simulink model "AUV_PM"  (R2020b)
settings: Solver=VariableStepAuto  StartTime=0.0  StopTime=10.0  RelTol=1e-3
InitFcn:
  | AUV_VehicleParameters
libraries: fl_lib x44, ee_lib x42, nesl_utility x33, AUVPropulsionSSC_lib x2
(part 1 of 2)
settings Model: DataDictionary=SignalInterfacesDD.sldd  Creator=jantonio  LastModifiedBy=jantonio

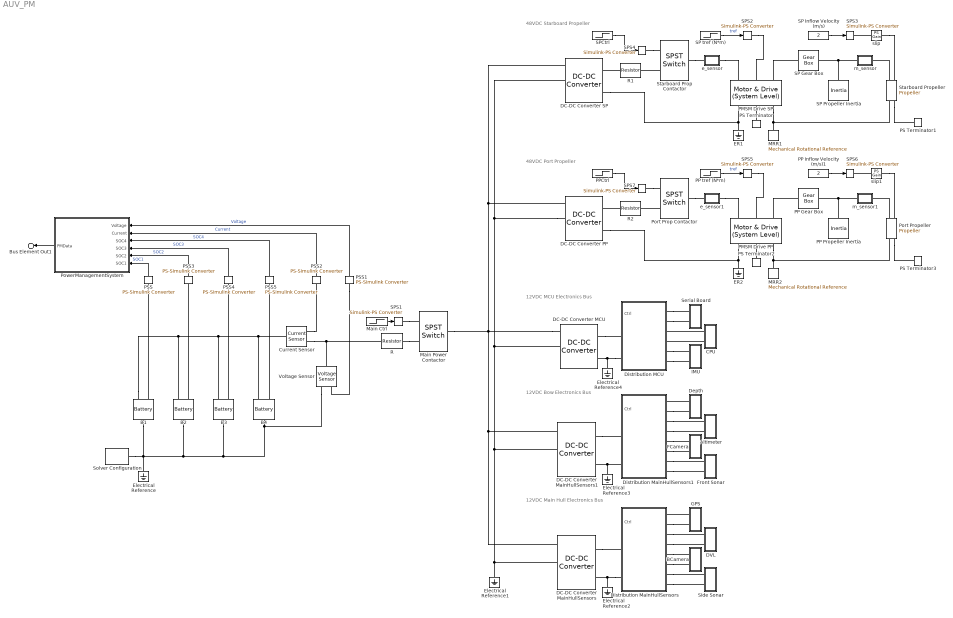
== system AUV_PM ==
  note: 12VDC Bow Electronics Bus
  note: 48VDC Port Propeller
  note: 12VDC MCU Electronics Bus
  note: 48VDC Starboard Propeller
  note: 12VDC Main Hull Electronics Bus
  Altimeter : Subsystem
  B{1..4} (4 alike) : ee_lib/Sources/Battery  Vnom=Vehicle.Battery.voltage V  prm_dir=1  R1_dis=2 Ohm  R1_ch=2 Ohm  R1=Vehicle.Battery.resistance Ohm  prm_AH=2  AH=Vehicle.Battery.capacity hr*A  V1=Vehicle.Battery.v1atAH1 V  AH1=Vehicle.Battery.AH1atV1 hr*A  prm_R2=1  R2=2000 Ohm  prm_dyn=2  Rp1=Vehicle.Battery.R1 Ohm  tau1=Vehicle.Battery.tau1 s  Rp2=0.005 Ohm  tau2=100 s  Rp3=0.005 Ohm  tau3=30 s  Rp4=0.005 Ohm  tau4=30 s  Rp5=0.005 Ohm  tau5=30 s  prm_fade=1  N_fade=100  AH_fade=45 hr*A  R1_fade=2.02 Ohm  R1_ch_fade=2.02 Ohm  V1_fade=10.35 V  i_specify=off  i_priority=None  i=0 A  i_nominal_specify=off  i_nominal_unit=A  i_nominal_value=1  v_specify=off  v_priority=None  v=0 V  v_nominal_specify=off  v_nominal_unit=V  v_nominal_value=1  charge_specify=on  charge_priority=High  charge=Vehicle.Battery.initcapacity hr*A  charge_nominal_specify=off  charge_nominal_unit=hr*A  charge_nominal_value=1  num_cycles_specify=off  num_cycles_priority=High  num_cycles=0  num_cycles_nominal_specify=off  num_cycles_nominal_unit=1  num_cycles_nominal_value=1  thermal_mass=30000 J/K  Tmeas=298.15 K  Vnom_T2=12 V  R1_T2=2.2 Ohm  R1_T2_dis=2.2 Ohm  R1_T2_ch=2.2 Ohm  V1_T2=11.4 V  R2_T2=2200 Ohm  Rp1_T2=0.005 Ohm  tau1_T2=30 s  Rp2_T2=0.005 Ohm  tau2_T2=30 s  Rp3_T2=0.005 Ohm  tau3_T2=30 s  Rp4_T2=0.005 Ohm  tau4_T2=30 s  Rp5_T2=0.005 Ohm  tau5_T2=30 s  Tmeas2=273.15 K  temperature_specify=off  temperature_priority=High  temperature=298.15 K  temperature_nominal_specify=off  temperature_nominal_unit=K  temperature_nominal_value=1
      settings: InternalSimscapePortConfiguration="{\"Bottom\":[],\"Left\":[{\"id\":\"p\",\"label\":\"+\",\"type\":\"foundation.electrical.electrical\"},{\"id\":\"q\",\"label\":\"q\",\"type\":\"output\"}],\"Right\":[{\"id\":\"n\",\"label\":\"-\",\"type\":\"foundation.electrical.electrical\"}],\"Top\":[]}"
  BCamera : Subsystem
  CPU : Subsystem
  Current Sensor : fl_lib/Electrical/Electrical Sensors/Current Sensor
  DC-DC Converter MCU : ee_lib/Semiconductors & Converters/Converters/DC-DC Converter  Vref_option=ee.enum.converters.voltageref.internal  v_ref=10 V  P_rated=10 W  droop_param=1  droop=0.1 V/A  droop_percent=2  reversible=0  efficiency=80  P_fixed=1 W  model_dynamics=0  tau=0.02 s  v_ini=10 V  G_diode=1e-8 1/Ohm  i1_max=2 A  fault_condition=1  fault_threshold=0.5  thermal_mass=100 J/K  initial_temperature=298.15 K
      settings: SourceProductBaseCode=PS  InternalSimscapePortConfiguration="{\"Bottom\":[],\"Left\":[{\"id\":\"p1\",\"label\":\"1+\",\"type\":\"foundation.electrical.electrical\"},{\"id\":\"n1\",\"label\":\"1-\",\"type\":\"foundation.electrical.electrical\"},{\"id\":\"F\",\"label\":\"F\",\"type\":\"input\"}],\"Right\":[{\"id\":\"p2\",\"label\":\"2+\",\"type\":\"foundation.electrical.electrical\"},{\"id\":\"n2\",\"label\":\"2-\",\"type\":\"foundation.electrical.electrical\"}],\"Top\":[]}"
  DC-DC Converter MainHullSensors : ee_lib/Semiconductors & Converters/Converters/DC-DC Converter  Vref_option=ee.enum.converters.voltageref.internal  v_ref=10 V  P_rated=10 W  droop_param=1  droop=0.1 V/A  droop_percent=2  reversible=0  efficiency=80  P_fixed=1 W  model_dynamics=0  tau=0.02 s  v_ini=10 V  G_diode=1e-8 1/Ohm  i1_max=2 A  fault_condition=1  fault_threshold=0.5  thermal_mass=100 J/K  initial_temperature=298.15 K
      settings: SourceProductBaseCode=PS  InternalSimscapePortConfiguration="{\"Bottom\":[],\"Left\":[{\"id\":\"p1\",\"label\":\"1+\",\"type\":\"foundation.electrical.electrical\"},{\"id\":\"n1\",\"label\":\"1-\",\"type\":\"foundation.electrical.electrical\"},{\"id\":\"F\",\"label\":\"F\",\"type\":\"input\"}],\"Right\":[{\"id\":\"p2\",\"label\":\"2+\",\"type\":\"foundation.electrical.electrical\"},{\"id\":\"n2\",\"label\":\"2-\",\"type\":\"foundation.electrical.electrical\"}],\"Top\":[]}"
  DC-DC Converter MainHullSensors1 : ee_lib/Semiconductors & Converters/Converters/DC-DC Converter  Vref_option=ee.enum.converters.voltageref.internal  v_ref=10 V  P_rated=10 W  droop_param=1  droop=0.1 V/A  droop_percent=2  reversible=0  efficiency=80  P_fixed=1 W  model_dynamics=0  tau=0.02 s  v_ini=10 V  G_diode=1e-8 1/Ohm  i1_max=2 A  fault_condition=1  fault_threshold=0.5  thermal_mass=100 J/K  initial_temperature=298.15 K
      settings: SourceProductBaseCode=PS  InternalSimscapePortConfiguration="{\"Bottom\":[],\"Left\":[{\"id\":\"p1\",\"label\":\"1+\",\"type\":\"foundation.electrical.electrical\"},{\"id\":\"n1\",\"label\":\"1-\",\"type\":\"foundation.electrical.electrical\"},{\"id\":\"F\",\"label\":\"F\",\"type\":\"input\"}],\"Right\":[{\"id\":\"p2\",\"label\":\"2+\",\"type\":\"foundation.electrical.electrical\"},{\"id\":\"n2\",\"label\":\"2-\",\"type\":\"foundation.electrical.electrical\"}],\"Top\":[]}"
  DC-DC Converter PP : ee_lib/Semiconductors & Converters/Converters/DC-DC Converter  Vref_option=ee.enum.converters.voltageref.internal  v_ref=10 V  P_rated=10 W  droop_param=1  droop=0.1 V/A  droop_percent=2  reversible=0  efficiency=80  P_fixed=1 W  model_dynamics=0  tau=0.02 s  v_ini=10 V  G_diode=1e-8 1/Ohm  i1_max=2 A  fault_condition=1  fault_threshold=0.5  thermal_mass=100 J/K  initial_temperature=298.15 K
      settings: SourceProductBaseCode=PS  InternalSimscapePortConfiguration="{\"Bottom\":[],\"Left\":[{\"id\":\"p1\",\"label\":\"1+\",\"type\":\"foundation.electrical.electrical\"},{\"id\":\"n1\",\"label\":\"1-\",\"type\":\"foundation.electrical.electrical\"},{\"id\":\"F\",\"label\":\"F\",\"type\":\"input\"}],\"Right\":[{\"id\":\"p2\",\"label\":\"2+\",\"type\":\"foundation.electrical.electrical\"},{\"id\":\"n2\",\"label\":\"2-\",\"type\":\"foundation.electrical.electrical\"}],\"Top\":[]}"
  DC-DC Converter SP : ee_lib/Semiconductors & Converters/Converters/DC-DC Converter  Vref_option=ee.enum.converters.voltageref.internal  v_ref=10 V  P_rated=10 W  droop_param=1  droop=0.1 V/A  droop_percent=2  reversible=0  efficiency=80  P_fixed=1 W  model_dynamics=0  tau=0.02 s  v_ini=10 V  G_diode=1e-8 1/Ohm  i1_max=2 A  fault_condition=1  fault_threshold=0.5  thermal_mass=100 J/K  initial_temperature=298.15 K
      settings: SourceProductBaseCode=PS  InternalSimscapePortConfiguration="{\"Bottom\":[],\"Left\":[{\"id\":\"p1\",\"label\":\"1+\",\"type\":\"foundation.electrical.electrical\"},{\"id\":\"n1\",\"label\":\"1-\",\"type\":\"foundation.electrical.electrical\"},{\"id\":\"F\",\"label\":\"F\",\"type\":\"input\"}],\"Right\":[{\"id\":\"p2\",\"label\":\"2+\",\"type\":\"foundation.electrical.electrical\"},{\"id\":\"n2\",\"label\":\"2-\",\"type\":\"foundation.electrical.electrical\"}],\"Top\":[]}"
  DVL : Subsystem
  Depth : Subsystem
  Distribution MCU : Subsystem
  Distribution MainHullSensors : Subsystem
  Distribution MainHullSensors1 : Subsystem
  ER1 : fl_lib/Electrical/Electrical Elements/Electrical Reference
      settings: SourceProductName=Foundation Library
  ER2 : fl_lib/Electrical/Electrical Elements/Electrical Reference
      settings: SourceProductName=Foundation Library
  Electrical Reference{,1..4} (5 alike) : fl_lib/Electrical/Electrical Elements/Electrical Reference
      settings: SourceProductBaseCode=MT,SS
  FCamera : Subsystem
  Front Sonar : Subsystem
  GPS : Subsystem
  IMU : Subsystem
  MRR1 : fl_lib/Mechanical/Rotational Elements/Mechanical Rotational Reference
  MRR2 : fl_lib/Mechanical/Rotational Elements/Mechanical Rotational Reference
  Main Ctrl : Step  Time=100  SampleTime=0
  Main Power Contactor : ee_lib/Switches & Breakers/SPST Switch  R_closed=0.01 Ohm  G_open=1e-6 S  Threshold=0.5 V  Width=0 V  model_dynamics=0  t_on=1e-3 s  t_off=1e-3 s  initial_vT=0 V
      settings: SourceProductBaseCode=PS  InternalSimscapePortConfiguration="{\"Bottom\":[],\"Left\":[{\"id\":\"vT\",\"label\":\"vT\",\"type\":\"input\"},{\"id\":\"p\",\"label\":\"\",\"type\":\"foundation.electrical.electrical\"}],\"Right\":[{\"id\":\"n\",\"label\":\"\",\"type\":\"foundation.electrical.electrical\"}],\"Top\":[]}"
  PMSM Drive PP : ee_lib/Electromechanical/Motor & Drive (System Level)  torque_speed_param=1  overtorque_param=ee.enum.electromech.overtorque.no  T_t=[0.991, 0.980, 0.270, 0] N*m  T_t_intermittent=[.36, .32, .28, 0] N*m  w_t=[0, 1200, 2950, 3600] rpm  torque_max=0.17 N*m  power_max=40 W  torque_max_intermittent=0.4 N*m  power_max_intermittent=120 W  time_overtorque=30 s  time_recover=60 s  Tc=1/(2*pi*500) s  losses_param=1  eff=95  w_eff=7000 deg/s  T_eff=0.13 N*m  Piron=0 W  Pbase=0 W  w_eff_vec=[-8000, -4000, 0, 4000, 8000] rpm  T_eff_vec=[0, .03, .06, .09] N*m  v_eff_vec=[100, 250, 400] V  losses_mat=[1.49, 1.67, 2.21, 3.1; .42, .69, 1.14, 2.03; .06, .24, .78, 1.68; .42, .69, 1.14, 2.03; 1.49, 1.67, 2.21, 3.1] W  efficiency_mat=[95, 95, 95, 95; 95, 95, 95, 95; 95, 95, 95, 95; 95, 95, 95, 95; 95, 95, 95, 95]  losses_mat_3D=ones(5, 4, 3) W  efficiency_mat_3D=95 * ones(5, 4, 3)  Res=1.16 Ohm  J=30 g*cm^2  lam=1e-4 N*m/(rad/s)  speed0=0 deg/s  faulted_specify=off  faulted_priority=None  faulted=0  faulted_nominal_specify=off  faulted_nominal_unit=1  faulted_nominal_value=1  torqueLimitContinuous_specify=off  torqueLimitContinuous_priority=None  torqueLimitContinuous=0 N*m  torqueLimitContinuous_nominal_specify=off  torqueLimitContinuous_nominal_unit=N*m  torqueLimitContinuous_nominal_value=1  alpha=3.93e-3 1/K  Tmeas=25 degC  Tmeas2=125 degC  losses_mat_T2=[1.49, 1.74, 2.49, 3.74; .42, .67, 1.42, 2.67; .06, .31, 1.06, 2.31; .42, .67, 1.42, 2.67; 1.49, 1.74, 2.49, 3.74] W  efficiency_mat_T2=[95, 95, 95, 95; 95, 95, 95, 95; 95, 95, 95, 95; 95, 95, 95, 95; 95, 95, 95, 95]  losses_mat_3D_T2=ones(5, 4, 3) W  efficiency_mat_3D_T2=95 * ones(5, 4, 3)  thermal_mass=100 J/K  initial_temperature=25 degC  fault_condition=1  fault_threshold=0.5
      settings: SourceProductBaseCode=PS  LogSimulationData=on
  PMSM Drive SP : ee_lib/Electromechanical/Motor & Drive (System Level)  torque_speed_param=1  overtorque_param=ee.enum.electromech.overtorque.no  T_t=[0.991, 0.980, 0.270, 0] N*m  T_t_intermittent=[.36, .32, .28, 0] N*m  w_t=[0, 1200, 2950, 3600] rpm  torque_max=0.17 N*m  power_max=40 W  torque_max_intermittent=0.4 N*m  power_max_intermittent=120 W  time_overtorque=30 s  time_recover=60 s  Tc=1/(2*pi*500) s  losses_param=1  eff=95  w_eff=7000 deg/s  T_eff=0.13 N*m  Piron=0 W  Pbase=0 W  w_eff_vec=[-8000, -4000, 0, 4000, 8000] rpm  T_eff_vec=[0, .03, .06, .09] N*m  v_eff_vec=[100, 250, 400] V  losses_mat=[1.49, 1.67, 2.21, 3.1; .42, .69, 1.14, 2.03; .06, .24, .78, 1.68; .42, .69, 1.14, 2.03; 1.49, 1.67, 2.21, 3.1] W  efficiency_mat=[95, 95, 95, 95; 95, 95, 95, 95; 95, 95, 95, 95; 95, 95, 95, 95; 95, 95, 95, 95]  losses_mat_3D=ones(5, 4, 3) W  efficiency_mat_3D=95 * ones(5, 4, 3)  Res=1.16 Ohm  J=30 g*cm^2  lam=1e-4 N*m/(rad/s)  speed0=0 deg/s  faulted_specify=off  faulted_priority=None  faulted=0  faulted_nominal_specify=off  faulted_nominal_unit=1  faulted_nominal_value=1  torqueLimitContinuous_specify=off  torqueLimitContinuous_priority=None  torqueLimitContinuous=0 N*m  torqueLimitContinuous_nominal_specify=off  torqueLimitContinuous_nominal_unit=N*m  torqueLimitContinuous_nominal_value=1  alpha=3.93e-3 1/K  Tmeas=25 degC  Tmeas2=125 degC  losses_mat_T2=[1.49, 1.74, 2.49, 3.74; .42, .67, 1.42, 2.67; .06, .31, 1.06, 2.31; .42, .67, 1.42, 2.67; 1.49, 1.74, 2.49, 3.74] W  efficiency_mat_T2=[95, 95, 95, 95; 95, 95, 95, 95; 95, 95, 95, 95; 95, 95, 95, 95; 95, 95, 95, 95]  losses_mat_3D_T2=ones(5, 4, 3) W  efficiency_mat_3D_T2=95 * ones(5, 4, 3)  thermal_mass=100 J/K  initial_temperature=25 degC  fault_condition=1  fault_threshold=0.5
      settings: SourceProductBaseCode=PS  LogSimulationData=on
  PP Propeller Inertia : fl_lib/Mechanical/Rotational Elements/Inertia  inertia=0.00015 kg*m^2  num_ports=foundation.enum.numPorts2.one  w_specify=off  w_priority=High  w=0 rad/s  w_nominal_specify=off  w_nominal_unit=rad/s  w_nominal_value=1  t_specify=off  t_priority=None  t=0 N*m  t_nominal_specify=off  t_nominal_unit=N*m  t_nominal_value=1
      settings: LogSimulationData=on
  PP Gear Box : fl_lib/Mechanical/Mechanisms/Gear Box  ratio=6  t_in_specify=off  t_in_priority=None  t_in=0 N*m  t_in_nominal_specify=off  t_in_nominal_unit=N*m  t_in_nominal_value=1  t_out_specify=off  t_out_priority=None  t_out=0 N*m  t_out_nominal_specify=off  t_out_nominal_unit=N*m  t_out_nominal_value=1
  PP Inflow Velocity (m/s)1 : Constant  Value=2
  PP tref (N*m) : Step  Time=0.05  Before=0.25  After=0.5  SampleTime=0
  PPCtrl : Step  Time=100  SampleTime=0
  PS Terminator{,1..3} (4 alike) : fl_lib/Physical Signals/Sinks/PS Terminator
  PSS{,3..5} (4 alike) : nesl_utility/PS-Simulink Converter  PhysicalDomain=network_engine_domain  SubClassName=ps_output  LeftPortType=input  RightPortType=output  PseudoPeriodic=off  Frequencies=[]  Unit=A*hr  AffineConversion=off
  PSS1 : nesl_utility/PS-Simulink Converter  PhysicalDomain=network_engine_domain  SubClassName=ps_output  LeftPortType=input  RightPortType=output  PseudoPeriodic=off  Frequencies=[]  Unit=inherit  AffineConversion=off
  PSS2 : nesl_utility/PS-Simulink Converter  PhysicalDomain=network_engine_domain  SubClassName=ps_output  LeftPortType=input  RightPortType=output  PseudoPeriodic=off  Frequencies=[]  Unit=A  AffineConversion=off
  Port Propeller : AUVPropulsionSSC_lib/Propeller  D=0.3 m  ktPoly="[0.0408   -0.2896   -0.1114    0.5420]"  kqPoly="[-0.0157   -0.0084   -0.0283    0.0947]"  rho=1027.3 kg/m^3  w_specify=off  w_priority=None  w=0 rad/s  w_nominal_specify=off  w_nominal_unit=rad/s  w_nominal_value=1  t_specify=off  t_priority=None  t=0 N*m  t_nominal_specify=off  t_nominal_unit=N*m  t_nominal_value=1
      settings: InternalSimscapePortConfiguration="{\"Bottom\":[],\"Left\":[{\"id\":\"Va\",\"label\":\"Va\",\"type\":\"input\"},{\"id\":\"R\",\"label\":\"R\",\"type\":\"foundation.mechanical.rotational.rotational\"}],\"Right\":[{\"id\":\"Thrust\",\"label\":\"Th\",\"type\":\"output\"},{\"id\":\"C\",\"label\":\"C\",\"type\":\"foundation.mechanical.rotational.rotational\"}],\"Top\":[]}"
  Port Prop Contactor : ee_lib/Switches & Breakers/SPST Switch  R_closed=0.01 Ohm  G_open=1e-6 S  Threshold=0.5 V  Width=0 V  model_dynamics=0  t_on=1e-3 s  t_off=1e-3 s  initial_vT=0 V
      settings: SourceProductBaseCode=PS  InternalSimscapePortConfiguration="{\"Bottom\":[],\"Left\":[{\"id\":\"vT\",\"label\":\"vT\",\"type\":\"input\"},{\"id\":\"p\",\"label\":\"\",\"type\":\"foundation.electrical.electrical\"}],\"Right\":[{\"id\":\"n\",\"label\":\"\",\"type\":\"foundation.electrical.electrical\"}],\"Top\":[]}"
  PowerManagementSystem : Subsystem
  R : ee_lib/Passive/Resistor  R=0.005 Ohm  R_tol=5  enable_R_tol=0  tol_distribution=1  nSigma=4  enable_operating_limits=0  operating_limit_action=2  max_working_voltage=100 V  power_rating=1 W  enable_faults=0  fault_action=1  R_faulted=inf Ohm  enable_temporal_fault=0  t_fault=1 s  enable_behavioral_fault=0  max_permissible_current=1 A  t_fail_on_current=1 s  noise_mode=0  sample_time=1e-3 s  repeatability=1  auto_seed=4111000739  user_seed=0  Tdevice=25 degC  alpha=3.93e-3 1/K  Tmeas=25 degC  thermal_mass=100 J/K  power_derating_T1=70 degC  power_derating_T2=155 degC  operating_temperature_range_vec=[-50, 150] degC  temperature_specify=off  temperature_priority=High  temperature=298.15 K  temperature_nominal_specify=off  temperature_nominal_unit=K  temperature_nominal_value=1
  R1 : ee_lib/Passive/Resistor  R=0.005 Ohm  R_tol=5  enable_R_tol=0  tol_distribution=1  nSigma=4  enable_operating_limits=0  operating_limit_action=2  max_working_voltage=100 V  power_rating=1 W  enable_faults=0  fault_action=1  R_faulted=inf Ohm  enable_temporal_fault=0  t_fault=1 s  enable_behavioral_fault=0  max_permissible_current=1 A  t_fail_on_current=1 s  noise_mode=0  sample_time=1e-3 s  repeatability=1  auto_seed=2084672538  user_seed=0  Tdevice=25 degC  alpha=3.93e-3 1/K  Tmeas=25 degC  thermal_mass=100 J/K  power_derating_T1=70 degC  power_derating_T2=155 degC  operating_temperature_range_vec=[-50, 150] degC  temperature_specify=off  temperature_priority=High  temperature=298.15 K  temperature_nominal_specify=off  temperature_nominal_unit=K  temperature_nominal_value=1
  R2 : ee_lib/Passive/Resistor  R=0.005 Ohm  R_tol=5  enable_R_tol=0  tol_distribution=1  nSigma=4  enable_operating_limits=0  operating_limit_action=2  max_working_voltage=100 V  power_rating=1 W  enable_faults=0  fault_action=1  R_faulted=inf Ohm  enable_temporal_fault=0  t_fault=1 s  enable_behavioral_fault=0  max_permissible_current=1 A  t_fail_on_current=1 s  noise_mode=0  sample_time=1e-3 s  repeatability=1  auto_seed=3437178441  user_seed=0  Tdevice=25 degC  alpha=3.93e-3 1/K  Tmeas=25 degC  thermal_mass=100 J/K  power_derating_T1=70 degC  power_derating_T2=155 degC  operating_temperature_range_vec=[-50, 150] degC  temperature_specify=off  temperature_priority=High  temperature=298.15 K  temperature_nominal_specify=off  temperature_nominal_unit=K  temperature_nominal_value=1
  SP Propeller Inertia : fl_lib/Mechanical/Rotational Elements/Inertia  inertia=0.00015 kg*m^2  num_ports=foundation.enum.numPorts2.one  w_specify=off  w_priority=High  w=0 rad/s  w_nominal_specify=off  w_nominal_unit=rad/s  w_nominal_value=1  t_specify=off  t_priority=None  t=0 N*m  t_nominal_specify=off  t_nominal_unit=N*m  t_nominal_value=1
      settings: LogSimulationData=on
  SP Gear Box : fl_lib/Mechanical/Mechanisms/Gear Box  ratio=6  t_in_specify=off  t_in_priority=None  t_in=0 N*m  t_in_nominal_specify=off  t_in_nominal_unit=N*m  t_in_nominal_value=1  t_out_specify=off  t_out_priority=None  t_out=0 N*m  t_out_nominal_specify=off  t_out_nominal_unit=N*m  t_out_nominal_value=1
  SP Inflow Velocity (m/s) : Constant  Value=2
  SP tref (N*m) : Step  Time=0.05  Before=0.25  After=0.5  SampleTime=0
  SPCtrl : Step  Time=100  SampleTime=0
  SPS1 : nesl_utility/Simulink-PS Converter  PhysicalDomain=network_engine_domain  SubClassName=ps_input  LeftPortType=input  RightPortType=output  PseudoPeriodic=off  Frequencies=[]  NoiseDistribution=none  NoiseParameters=[]  Unit=1  AffineConversion=off  FilteringAndDerivatives=provide  SimscapeFilterOrder=1  InputFilterTimeConstant=0.001  UdotUserProvided=0
      settings: SourceProductBaseCode=MT,SS
  SPS2 : nesl_utility/Simulink-PS Converter  PhysicalDomain=network_engine_domain  SubClassName=ps_input  LeftPortType=input  RightPortType=output  PseudoPeriodic=off  Frequencies=[]  NoiseDistribution=none  NoiseParameters=[]  Unit=N*m  AffineConversion=off  FilteringAndDerivatives=provide  SimscapeFilterOrder=1  InputFilterTimeConstant=0.001  UdotUserProvided=0
  SPS3 : nesl_utility/Simulink-PS Converter  PhysicalDomain=network_engine_domain  SubClassName=ps_input  LeftPortType=input  RightPortType=output  PseudoPeriodic=off  Frequencies=[]  NoiseDistribution=none  NoiseParameters=[]  Unit=m/s  AffineConversion=off  FilteringAndDerivatives=provide  SimscapeFilterOrder=1  InputFilterTimeConstant=0.001  UdotUserProvided=0
  SPS4 : nesl_utility/Simulink-PS Converter  PhysicalDomain=network_engine_domain  SubClassName=ps_input  LeftPortType=input  RightPortType=output  PseudoPeriodic=off  Frequencies=[]  NoiseDistribution=none  NoiseParameters=[]  Unit=1  AffineConversion=off  FilteringAndDerivatives=provide  SimscapeFilterOrder=1  InputFilterTimeConstant=0.001  UdotUserProvided=0
      settings: SourceProductBaseCode=MT,SS
  SPS5 : nesl_utility/Simulink-PS Converter  PhysicalDomain=network_engine_domain  SubClassName=ps_input  LeftPortType=input  RightPortType=output  PseudoPeriodic=off  Frequencies=[]  NoiseDistribution=none  NoiseParameters=[]  Unit=N*m  AffineConversion=off  FilteringAndDerivatives=provide  SimscapeFilterOrder=1  InputFilterTimeConstant=0.001  UdotUserProvided=0
  SPS6 : nesl_utility/Simulink-PS Converter  PhysicalDomain=network_engine_domain  SubClassName=ps_input  LeftPortType=input  RightPortType=output  PseudoPeriodic=off  Frequencies=[]  NoiseDistribution=none  NoiseParameters=[]  Unit=m/s  AffineConversion=off  FilteringAndDerivatives=provide  SimscapeFilterOrder=1  InputFilterTimeConstant=0.001  UdotUserProvided=0
  SPS7 : nesl_utility/Simulink-PS Converter  PhysicalDomain=network_engine_domain  SubClassName=ps_input  LeftPortType=input  RightPortType=output  PseudoPeriodic=off  Frequencies=[]  NoiseDistribution=none  NoiseParameters=[]  Unit=1  AffineConversion=off  FilteringAndDerivatives=provide  SimscapeFilterOrder=1  InputFilterTimeConstant=0.001  UdotUserProvided=0
      settings: SourceProductBaseCode=MT,SS
  Serial Board : Subsystem
  Side Sonar : Subsystem
  Solver Configuration : nesl_utility/Solver Configuration  PhysicalDomain=network_engine_domain  SubClassName=solver  LeftPortType=input  RightPortType=generic  Tones=[]  Harmonics=[]  SimulateNoise=off  Profile=off  UseLocalSampling=off  EnableSwitchedLinearOptims=on  FrequencyDomain=off  UseCCode=off  RelTol=0.001  AbsTol=1e-06  MinStep=1e-09  ToWorkspace=off  RevertToSquareIcSolve=off  NumHomotopyIterations=100  PhasorMode=off  PhasorModeNumHarmonics=1  DoDC=off  ResidualTolerance=1e-09  UseLocalSolver=off  LocalSolverChoice=NE_BACKWARD_EULER_ADVANCER  LocalSolverSampleTime=0.001  DoFixedCost=off  MaxNonlinIter=3  MaxModeIter=2  ComputeImpulses=off  ImpulseIterations=2  LinearAlgebra=auto  EquationFormulation=NE_TIME_EF  DelaysMemoryBudget=1024  AutomaticFiltering=on  FilteringTimeConstant=0.001  PartitionStorageMethod=AS_NEEDED  PartitionMemoryBudget=1024  PartitionMethod=ROBUST
      settings: SourceProductBaseCode=MT,SS
  Starboard Propeller : AUVPropulsionSSC_lib/Propeller  D=0.3 m  ktPoly="[0.0408   -0.2896   -0.1114    0.5420]"  kqPoly="[-0.0157   -0.0084   -0.0283    0.0947]"  rho=1027.3 kg/m^3  w_specify=off  w_priority=None  w=0 rad/s  w_nominal_specify=off  w_nominal_unit=rad/s  w_nominal_value=1  t_specify=off  t_priority=None  t=0 N*m  t_nominal_specify=off  t_nominal_unit=N*m  t_nominal_value=1
      settings: InternalSimscapePortConfiguration="{\"Bottom\":[],\"Left\":[{\"id\":\"Va\",\"label\":\"Va\",\"type\":\"input\"},{\"id\":\"R\",\"label\":\"R\",\"type\":\"foundation.mechanical.rotational.rotational\"}],\"Right\":[{\"id\":\"Thrust\",\"label\":\"Th\",\"type\":\"output\"},{\"id\":\"C\",\"label\":\"C\",\"type\":\"foundation.mechanical.rotational.rotational\"}],\"Top\":[]}"
  Starboard Prop Contactor : ee_lib/Switches & Breakers/SPST Switch  R_closed=0.01 Ohm  G_open=1e-6 S  Threshold=0.5 V  Width=0 V  model_dynamics=0  t_on=1e-3 s  t_off=1e-3 s  initial_vT=0 V
      settings: SourceProductBaseCode=PS  InternalSimscapePortConfiguration="{\"Bottom\":[],\"Left\":[{\"id\":\"vT\",\"label\":\"vT\",\"type\":\"input\"},{\"id\":\"p\",\"label\":\"\",\"type\":\"foundation.electrical.electrical\"}],\"Right\":[{\"id\":\"n\",\"label\":\"\",\"type\":\"foundation.electrical.electrical\"}],\"Top\":[]}"
  Voltage Sensor : fl_lib/Electrical/Electrical Sensors/Voltage Sensor
  e_sensor : Subsystem
  e_sensor1 : Subsystem
  m_sensor : Subsystem
  m_sensor1 : Subsystem
  slip : fl_lib/Physical Signals/Functions/PS Gain  gain=1
  slip1 : fl_lib/Physical Signals/Functions/PS Gain  gain=1
  Bus Element Out1 : Outport  PortName=PMData
  wires:
  PowerManagementSystem/1(PMData) -> Bus Element Out1/1
  PSS/1 -> PowerManagementSystem/6(SOC1)  "SOC1"
  SPCtrl/1 -> SPS4/1
  PSS1/1 -> PowerManagementSystem/1(Voltage)  "Voltage"
  Main Ctrl/1 -> SPS1/1
  PSS5/1 -> PowerManagementSystem/3(SOC4)  "SOC4"
  PP Inflow Velocity (m/s)1/1 -> SPS6/1
  PPCtrl/1 -> SPS7/1
  PSS2/1 -> PowerManagementSystem/2(Current)  "Current"
  SP tref (N*m)/1 -> SPS2/1  "tref"
  PP tref (N*m)/1 -> SPS5/1  "tref"
  SP Inflow Velocity (m/s)/1 -> SPS3/1
  PSS3/1 -> PowerManagementSystem/5(SOC2)  "SOC2"
  PSS4/1 -> PowerManagementSystem/4(SOC3)  "SOC3"
  connections:
  B1/LConn1 -- B2/LConn1 -- B3/LConn1 -- Current Sensor/LConn1 -- B4/LConn1
  DC-DC Converter PP/LConn2 -- DC-DC Converter SP/LConn2 -- DC-DC Converter MCU/LConn2 -- Electrical Reference1/LConn1 -- DC-DC Converter MainHullSensors/LConn2 -- DC-DC Converter MainHullSensors1/LConn2
  Current Sensor/RConn2 -- R/RConn1 -- Voltage Sensor/LConn1
  PMSM Drive SP/RConn1 -- DC-DC Converter SP/RConn2 -- ER1/LConn1
  B2/RConn1 -- B1/RConn1 -- Solver Configuration/RConn1 -- Electrical Reference/LConn1 -- B4/RConn1 -- Voltage Sensor/RConn2 -- B3/RConn1
  SP Gear Box/RConn1 -- SP Propeller Inertia/LConn1 -- m_sensor/LConn1
  Distribution MCU/LConn2 -- DC-DC Converter MCU/RConn2 -- Electrical Reference4/LConn1
  Distribution MainHullSensors/LConn2 -- Electrical Reference2/LConn1 -- DC-DC Converter MainHullSensors/RConn2
  DC-DC Converter MCU/LConn1 -- Main Power Contactor/RConn1 -- DC-DC Converter SP/LConn1 -- DC-DC Converter PP/LConn1 -- DC-DC Converter MainHullSensors1/LConn1 -- DC-DC Converter MainHullSensors/LConn1
  PMSM Drive PP/RConn1 -- ER2/LConn1 -- DC-DC Converter PP/RConn2
  DC-DC Converter MainHullSensors1/RConn2 -- Electrical Reference3/LConn1 -- Distribution MainHullSensors1/LConn2
  Starboard Propeller/RConn2 -- PMSM Drive SP/RConn3 -- MRR1/LConn1
  MRR2/LConn1 -- PMSM Drive PP/RConn3 -- Port Propeller/RConn2
  PP Gear Box/RConn1 -- m_sensor1/LConn1 -- PP Propeller Inertia/LConn1
  SPS2/RConn1 -- PMSM Drive SP/LConn2
  Distribution MainHullSensors/RConn7 -- Side Sonar/LConn1
  B2/LConn2 -- PSS3/LConn1
  B4/LConn2 -- PSS5/LConn1
  Distribution MCU/RConn5 -- IMU/LConn1
  Distribution MainHullSensors/RConn5 -- BCamera/LConn1
  SPS1/RConn1 -- Main Power Contactor/LConn1
  PSS/LConn1 -- B1/LConn2
  Distribution MainHullSensors1/RConn3 -- Altimeter/LConn1
  PSS1/LConn1 -- Voltage Sensor/RConn1
  SP Gear Box/LConn1 -- PMSM Drive SP/LConn3
  B3/LConn2 -- PSS4/LConn1
  Starboard Prop Contactor/LConn2 -- R1/RConn1
  Depth/LConn1 -- Distribution MainHullSensors1/RConn1
  Starboard Propeller/LConn2 -- m_sensor/RConn1
  e_sensor/RConn1 -- PMSM Drive SP/LConn1
  Distribution MainHullSensors1/RConn5 -- FCamera/LConn1
  Distribution MainHullSensors1/RConn8 -- Front Sonar/LConn2
  Distribution MainHullSensors1/RConn6 -- FCamera/LConn2
  Distribution MainHullSensors/RConn3 -- DVL/LConn1
  Distribution MainHullSensors1/RConn4 -- Altimeter/LConn2
  SPS7/RConn1 -- Port Prop Contactor/LConn1
  PS Terminator/LConn1 -- PMSM Drive SP/RConn2
  Distribution MCU/RConn1 -- Serial Board/LConn1
  Distribution MainHullSensors/RConn6 -- BCamera/LConn2
  PP Gear Box/LConn1 -- PMSM Drive PP/LConn3
  Current Sensor/RConn1 -- PSS2/LConn1
  SPS5/RConn1 -- PMSM Drive PP/LConn2
  Distribution MCU/RConn6 -- IMU/LConn2
  DC-DC Converter MainHullSensors1/RConn1 -- Distribution MainHullSensors1/LConn1
  Distribution MainHullSensors/RConn4 -- DVL/LConn2
  PS Terminator2/LConn1 -- PMSM Drive PP/RConn2
  slip1/RConn1 -- Port Propeller/LConn1
  Port Prop Contactor/LConn2 -- R2/RConn1
  R1/LConn1 -- DC-DC Converter SP/RConn1
  R/LConn1 -- Main Power Contactor/LConn2
  R2/LConn1 -- DC-DC Converter PP/RConn1
  Starboard Propeller/RConn1 -- PS Terminator1/LConn1
  Distribution MainHullSensors1/RConn7 -- Front Sonar/LConn1
  e_sensor1/RConn1 -- PMSM Drive PP/LConn1
  DC-DC Converter MainHullSensors/RConn1 -- Distribution MainHullSensors/LConn1
  Distribution MainHullSensors/RConn8 -- Side Sonar/LConn2
  Distribution MCU/RConn2 -- Serial Board/LConn2
  slip1/LConn1 -- SPS6/RConn1
  CPU/LConn2 -- Distribution MCU/RConn4
  slip/LConn1 -- SPS3/RConn1
  slip/RConn1 -- Starboard Propeller/LConn1
  GPS/LConn1 -- Distribution MainHullSensors/RConn1
  DC-DC Converter MCU/RConn1 -- Distribution MCU/LConn1
  Port Prop Contactor/RConn1 -- e_sensor1/LConn1
  Starboard Prop Contactor/RConn1 -- e_sensor/LConn1
  SPS4/RConn1 -- Starboard Prop Contactor/LConn1
  Distribution MainHullSensors1/RConn2 -- Depth/LConn2
  Port Propeller/RConn1 -- PS Terminator3/LConn1
  Distribution MainHullSensors/RConn2 -- GPS/LConn2
  Port Propeller/LConn2 -- m_sensor1/RConn1
  CPU/LConn1 -- Distribution MCU/RConn3

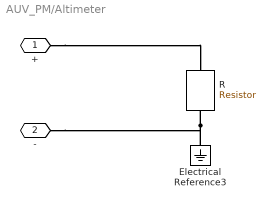
== system AUV_PM/Altimeter ==
  Electrical Reference3 : fl_lib/Electrical/Electrical Elements/Electrical Reference
      settings: SourceProductBaseCode=MT,SS
  R : ee_lib/Passive/Resistor  R=5 Ohm  R_tol=5  enable_R_tol=0  tol_distribution=1  nSigma=4  enable_operating_limits=0  operating_limit_action=2  max_working_voltage=100 V  power_rating=1 W  enable_faults=0  fault_action=1  R_faulted=inf Ohm  enable_temporal_fault=0  t_fault=1 s  enable_behavioral_fault=0  max_permissible_current=1 A  t_fail_on_current=1 s  noise_mode=0  sample_time=1e-3 s  repeatability=1  auto_seed=3499211588  user_seed=0  Tdevice=25 degC  alpha=3.93e-3 1/K  Tmeas=25 degC  thermal_mass=100 J/K  power_derating_T1=70 degC  power_derating_T2=155 degC  operating_temperature_range_vec=[-50, 150] degC  temperature_specify=off  temperature_priority=High  temperature=298.15 K  temperature_nominal_specify=off  temperature_nominal_unit=K  temperature_nominal_value=1
  + : PMIOPort  Side=Left
  - : PMIOPort  Port=2  Side=Left
  connections:
  +/RConn1 -- R/LConn1
  R/RConn1 -- Electrical Reference3/LConn1 -- -/RConn1

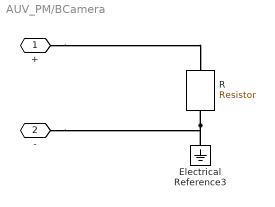
== system AUV_PM/BCamera ==
  Electrical Reference3 : fl_lib/Electrical/Electrical Elements/Electrical Reference
      settings: SourceProductBaseCode=MT,SS
  R : ee_lib/Passive/Resistor  R=5 Ohm  R_tol=5  enable_R_tol=0  tol_distribution=1  nSigma=4  enable_operating_limits=0  operating_limit_action=2  max_working_voltage=100 V  power_rating=1 W  enable_faults=0  fault_action=1  R_faulted=inf Ohm  enable_temporal_fault=0  t_fault=1 s  enable_behavioral_fault=0  max_permissible_current=1 A  t_fail_on_current=1 s  noise_mode=0  sample_time=1e-3 s  repeatability=1  auto_seed=3890346746  user_seed=0  Tdevice=25 degC  alpha=3.93e-3 1/K  Tmeas=25 degC  thermal_mass=100 J/K  power_derating_T1=70 degC  power_derating_T2=155 degC  operating_temperature_range_vec=[-50, 150] degC  temperature_specify=off  temperature_priority=High  temperature=298.15 K  temperature_nominal_specify=off  temperature_nominal_unit=K  temperature_nominal_value=1
  + : PMIOPort  Side=Left
  - : PMIOPort  Port=2  Side=Left
  connections:
  +/RConn1 -- R/LConn1
  R/RConn1 -- Electrical Reference3/LConn1 -- -/RConn1

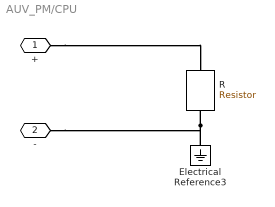
== system AUV_PM/CPU ==
  Electrical Reference3 : fl_lib/Electrical/Electrical Elements/Electrical Reference
      settings: SourceProductBaseCode=MT,SS
  R : ee_lib/Passive/Resistor  R=5 Ohm  R_tol=5  enable_R_tol=0  tol_distribution=1  nSigma=4  enable_operating_limits=0  operating_limit_action=2  max_working_voltage=100 V  power_rating=1 W  enable_faults=0  fault_action=1  R_faulted=inf Ohm  enable_temporal_fault=0  t_fault=1 s  enable_behavioral_fault=0  max_permissible_current=1 A  t_fail_on_current=1 s  noise_mode=0  sample_time=1e-3 s  repeatability=1  auto_seed=545404223  user_seed=0  Tdevice=25 degC  alpha=3.93e-3 1/K  Tmeas=25 degC  thermal_mass=100 J/K  power_derating_T1=70 degC  power_derating_T2=155 degC  operating_temperature_range_vec=[-50, 150] degC  temperature_specify=off  temperature_priority=High  temperature=298.15 K  temperature_nominal_specify=off  temperature_nominal_unit=K  temperature_nominal_value=1
  + : PMIOPort  Side=Left
  - : PMIOPort  Port=2  Side=Left
  connections:
  +/RConn1 -- R/LConn1
  R/RConn1 -- Electrical Reference3/LConn1 -- -/RConn1

== system AUV_PM/DVL ==
  Electrical Reference3 : fl_lib/Electrical/Electrical Elements/Electrical Reference
      settings: SourceProductBaseCode=MT,SS
  R : ee_lib/Passive/Resistor  R=5 Ohm  R_tol=5  enable_R_tol=0  tol_distribution=1  nSigma=4  enable_operating_limits=0  operating_limit_action=2  max_working_voltage=100 V  power_rating=1 W  enable_faults=0  fault_action=1  R_faulted=inf Ohm  enable_temporal_fault=0  t_fault=1 s  enable_behavioral_fault=0  max_permissible_current=1 A  t_fail_on_current=1 s  noise_mode=0  sample_time=1e-3 s  repeatability=1  auto_seed=3922919431  user_seed=0  Tdevice=25 degC  alpha=3.93e-3 1/K  Tmeas=25 degC  thermal_mass=100 J/K  power_derating_T1=70 degC  power_derating_T2=155 degC  operating_temperature_range_vec=[-50, 150] degC  temperature_specify=off  temperature_priority=High  temperature=298.15 K  temperature_nominal_specify=off  temperature_nominal_unit=K  temperature_nominal_value=1
  + : PMIOPort  Side=Left
  - : PMIOPort  Port=2  Side=Left
  connections:
  -/RConn1 -- Electrical Reference3/LConn1 -- R/RConn1
  +/RConn1 -- R/LConn1

== system AUV_PM/Depth ==
  Electrical Reference3 : fl_lib/Electrical/Electrical Elements/Electrical Reference
      settings: SourceProductBaseCode=MT,SS
  R : ee_lib/Passive/Resistor  R=5 Ohm  R_tol=5  enable_R_tol=0  tol_distribution=1  nSigma=4  enable_operating_limits=0  operating_limit_action=2  max_working_voltage=100 V  power_rating=1 W  enable_faults=0  fault_action=1  R_faulted=inf Ohm  enable_temporal_fault=0  t_fault=1 s  enable_behavioral_fault=0  max_permissible_current=1 A  t_fail_on_current=1 s  noise_mode=0  sample_time=1e-3 s  repeatability=1  auto_seed=2715962282  user_seed=0  Tdevice=25 degC  alpha=3.93e-3 1/K  Tmeas=25 degC  thermal_mass=100 J/K  power_derating_T1=70 degC  power_derating_T2=155 degC  operating_temperature_range_vec=[-50, 150] degC  temperature_specify=off  temperature_priority=High  temperature=298.15 K  temperature_nominal_specify=off  temperature_nominal_unit=K  temperature_nominal_value=1
  + : PMIOPort  Side=Left
  - : PMIOPort  Port=2  Side=Left
  connections:
  -/RConn1 -- Electrical Reference3/LConn1 -- R/RConn1
  +/RConn1 -- R/LConn1

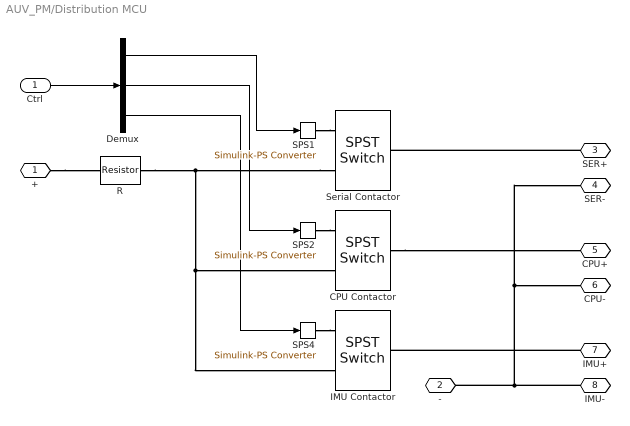
== system AUV_PM/Distribution MCU ==
  Ctrl : Inport
  CPU Contactor : ee_lib/Switches & Breakers/SPST Switch  R_closed=0.005 Ohm  G_open=1e-6 S  Threshold=0.5 V  Width=0 V  model_dynamics=0  t_on=1e-3 s  t_off=1e-3 s  initial_vT=0 V
      settings: SourceProductBaseCode=PS  InternalSimscapePortConfiguration="{\"Bottom\":[],\"Left\":[{\"id\":\"vT\",\"label\":\"vT\",\"type\":\"input\"},{\"id\":\"p\",\"label\":\"\",\"type\":\"foundation.electrical.electrical\"}],\"Right\":[{\"id\":\"n\",\"label\":\"\",\"type\":\"foundation.electrical.electrical\"}],\"Top\":[]}"
  Demux : Demux  Outputs=3
  IMU Contactor : ee_lib/Switches & Breakers/SPST Switch  R_closed=0.005 Ohm  G_open=1e-6 S  Threshold=0.5 V  Width=0 V  model_dynamics=0  t_on=1e-3 s  t_off=1e-3 s  initial_vT=0 V
      settings: SourceProductBaseCode=PS  InternalSimscapePortConfiguration="{\"Bottom\":[],\"Left\":[{\"id\":\"vT\",\"label\":\"vT\",\"type\":\"input\"},{\"id\":\"p\",\"label\":\"\",\"type\":\"foundation.electrical.electrical\"}],\"Right\":[{\"id\":\"n\",\"label\":\"\",\"type\":\"foundation.electrical.electrical\"}],\"Top\":[]}"
  R : ee_lib/Passive/Resistor  R=0.005 Ohm  R_tol=5  enable_R_tol=0  tol_distribution=1  nSigma=4  enable_operating_limits=0  operating_limit_action=2  max_working_voltage=100 V  power_rating=1 W  enable_faults=0  fault_action=1  R_faulted=inf Ohm  enable_temporal_fault=0  t_fault=1 s  enable_behavioral_fault=0  max_permissible_current=1 A  t_fail_on_current=1 s  noise_mode=0  sample_time=1e-3 s  repeatability=1  auto_seed=418932850  user_seed=0  Tdevice=25 degC  alpha=3.93e-3 1/K  Tmeas=25 degC  thermal_mass=100 J/K  power_derating_T1=70 degC  power_derating_T2=155 degC  operating_temperature_range_vec=[-50, 150] degC  temperature_specify=off  temperature_priority=High  temperature=298.15 K  temperature_nominal_specify=off  temperature_nominal_unit=K  temperature_nominal_value=1
  SPS1 : nesl_utility/Simulink-PS Converter  PhysicalDomain=network_engine_domain  SubClassName=ps_input  LeftPortType=input  RightPortType=output  PseudoPeriodic=off  Frequencies=[]  NoiseDistribution=none  NoiseParameters=[]  Unit=1  AffineConversion=off  FilteringAndDerivatives=provide  SimscapeFilterOrder=1  InputFilterTimeConstant=0.001  UdotUserProvided=0
  SPS2 : nesl_utility/Simulink-PS Converter  PhysicalDomain=network_engine_domain  SubClassName=ps_input  LeftPortType=input  RightPortType=output  PseudoPeriodic=off  Frequencies=[]  NoiseDistribution=none  NoiseParameters=[]  Unit=1  AffineConversion=off  FilteringAndDerivatives=provide  SimscapeFilterOrder=1  InputFilterTimeConstant=0.001  UdotUserProvided=0
  SPS4 : nesl_utility/Simulink-PS Converter  PhysicalDomain=network_engine_domain  SubClassName=ps_input  LeftPortType=input  RightPortType=output  PseudoPeriodic=off  Frequencies=[]  NoiseDistribution=none  NoiseParameters=[]  Unit=1  AffineConversion=off  FilteringAndDerivatives=provide  SimscapeFilterOrder=1  InputFilterTimeConstant=0.001  UdotUserProvided=0
  Serial Contactor : ee_lib/Switches & Breakers/SPST Switch  R_closed=0.005 Ohm  G_open=1e-6 S  Threshold=0.5 V  Width=0 V  model_dynamics=0  t_on=1e-3 s  t_off=1e-3 s  initial_vT=0 V
      settings: SourceProductBaseCode=PS  InternalSimscapePortConfiguration="{\"Bottom\":[],\"Left\":[{\"id\":\"vT\",\"label\":\"vT\",\"type\":\"input\"},{\"id\":\"p\",\"label\":\"\",\"type\":\"foundation.electrical.electrical\"}],\"Right\":[{\"id\":\"n\",\"label\":\"\",\"type\":\"foundation.electrical.electrical\"}],\"Top\":[]}"
  + : PMIOPort  Side=Left
  - : PMIOPort  Port=2  Side=Left
  SER+ : PMIOPort  Port=3  Side=Right
  SER- : PMIOPort  Port=4  Side=Right
  CPU+ : PMIOPort  Port=5  Side=Right
  CPU- : PMIOPort  Port=6  Side=Right
  IMU+ : PMIOPort  Port=7  Side=Right
  IMU- : PMIOPort  Port=8  Side=Right
  wires:
  Ctrl/1 -> Demux/1
  Demux/1 -> SPS1/1
  Demux/2 -> SPS2/1
  Demux/3 -> SPS4/1
  connections:
  SPS4/RConn1 -- IMU Contactor/LConn1
  SPS2/RConn1 -- CPU Contactor/LConn1
  SPS1/RConn1 -- Serial Contactor/LConn1
  CPU Contactor/RConn1 -- CPU+/RConn1
  SER+/RConn1 -- Serial Contactor/RConn1
  IMU+/RConn1 -- IMU Contactor/RConn1
  +/RConn1 -- R/LConn1
  Serial Contactor/LConn2 -- R/RConn1 -- IMU Contactor/LConn2 -- CPU Contactor/LConn2
  IMU-/RConn1 -- SER-/RConn1 -- CPU-/RConn1 -- -/RConn1

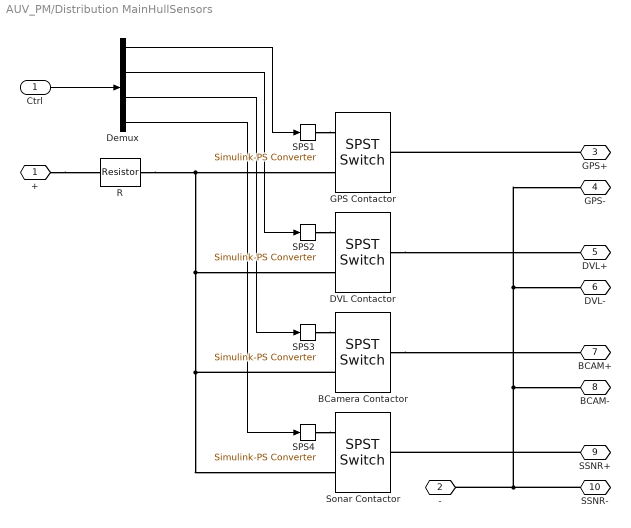
== system AUV_PM/Distribution MainHullSensors ==
  Ctrl : Inport
  BCamera Contactor : ee_lib/Switches & Breakers/SPST Switch  R_closed=0.005 Ohm  G_open=1e-6 S  Threshold=0.5 V  Width=0 V  model_dynamics=0  t_on=1e-3 s  t_off=1e-3 s  initial_vT=0 V
      settings: SourceProductBaseCode=PS  InternalSimscapePortConfiguration="{\"Bottom\":[],\"Left\":[{\"id\":\"vT\",\"label\":\"vT\",\"type\":\"input\"},{\"id\":\"p\",\"label\":\"\",\"type\":\"foundation.electrical.electrical\"}],\"Right\":[{\"id\":\"n\",\"label\":\"\",\"type\":\"foundation.electrical.electrical\"}],\"Top\":[]}"
  DVL Contactor : ee_lib/Switches & Breakers/SPST Switch  R_closed=0.005 Ohm  G_open=1e-6 S  Threshold=0.5 V  Width=0 V  model_dynamics=0  t_on=1e-3 s  t_off=1e-3 s  initial_vT=0 V
      settings: SourceProductBaseCode=PS  InternalSimscapePortConfiguration="{\"Bottom\":[],\"Left\":[{\"id\":\"vT\",\"label\":\"vT\",\"type\":\"input\"},{\"id\":\"p\",\"label\":\"\",\"type\":\"foundation.electrical.electrical\"}],\"Right\":[{\"id\":\"n\",\"label\":\"\",\"type\":\"foundation.electrical.electrical\"}],\"Top\":[]}"
  Demux : Demux
  GPS Contactor : ee_lib/Switches & Breakers/SPST Switch  R_closed=0.005 Ohm  G_open=1e-6 S  Threshold=0.5 V  Width=0 V  model_dynamics=0  t_on=1e-3 s  t_off=1e-3 s  initial_vT=0 V
      settings: SourceProductBaseCode=PS  InternalSimscapePortConfiguration="{\"Bottom\":[],\"Left\":[{\"id\":\"vT\",\"label\":\"vT\",\"type\":\"input\"},{\"id\":\"p\",\"label\":\"\",\"type\":\"foundation.electrical.electrical\"}],\"Right\":[{\"id\":\"n\",\"label\":\"\",\"type\":\"foundation.electrical.electrical\"}],\"Top\":[]}"
  R : ee_lib/Passive/Resistor  R=0.005 Ohm  R_tol=5  enable_R_tol=0  tol_distribution=1  nSigma=4  enable_operating_limits=0  operating_limit_action=2  max_working_voltage=100 V  power_rating=1 W  enable_faults=0  fault_action=1  R_faulted=inf Ohm  enable_temporal_fault=0  t_fault=1 s  enable_behavioral_fault=0  max_permissible_current=1 A  t_fail_on_current=1 s  noise_mode=0  sample_time=1e-3 s  repeatability=1  auto_seed=1196140742  user_seed=0  Tdevice=25 degC  alpha=3.93e-3 1/K  Tmeas=25 degC  thermal_mass=100 J/K  power_derating_T1=70 degC  power_derating_T2=155 degC  operating_temperature_range_vec=[-50, 150] degC  temperature_specify=off  temperature_priority=High  temperature=298.15 K  temperature_nominal_specify=off  temperature_nominal_unit=K  temperature_nominal_value=1
  SPS{1..4} (4 alike) : nesl_utility/Simulink-PS Converter  PhysicalDomain=network_engine_domain  SubClassName=ps_input  LeftPortType=input  RightPortType=output  PseudoPeriodic=off  Frequencies=[]  NoiseDistribution=none  NoiseParameters=[]  Unit=1  AffineConversion=off  FilteringAndDerivatives=provide  SimscapeFilterOrder=1  InputFilterTimeConstant=0.001  UdotUserProvided=0
  Sonar Contactor : ee_lib/Switches & Breakers/SPST Switch  R_closed=0.005 Ohm  G_open=1e-6 S  Threshold=0.5 V  Width=0 V  model_dynamics=0  t_on=1e-3 s  t_off=1e-3 s  initial_vT=0 V
      settings: SourceProductBaseCode=PS  InternalSimscapePortConfiguration="{\"Bottom\":[],\"Left\":[{\"id\":\"vT\",\"label\":\"vT\",\"type\":\"input\"},{\"id\":\"p\",\"label\":\"\",\"type\":\"foundation.electrical.electrical\"}],\"Right\":[{\"id\":\"n\",\"label\":\"\",\"type\":\"foundation.electrical.electrical\"}],\"Top\":[]}"
  + : PMIOPort  Side=Left
  - : PMIOPort  Port=2  Side=Left
  GPS+ : PMIOPort  Port=3  Side=Right
  GPS- : PMIOPort  Port=4  Side=Right
  DVL+ : PMIOPort  Port=5  Side=Right
  DVL- : PMIOPort  Port=6  Side=Right
  BCAM+ : PMIOPort  Port=7  Side=Right
  BCAM- : PMIOPort  Port=8  Side=Right
  SSNR+ : PMIOPort  Port=9  Side=Right
  SSNR- : PMIOPort  Port=10  Side=Right
  wires:
  Demux/4 -> SPS4/1
  Demux/3 -> SPS3/1
  Demux/2 -> SPS2/1
  Demux/1 -> SPS1/1
  Ctrl/1 -> Demux/1
  connections:
  R/RConn1 -- GPS Contactor/LConn2 -- DVL Contactor/LConn2 -- Sonar Contactor/LConn2 -- BCamera Contactor/LConn2
  +/RConn1 -- R/LConn1
  SSNR-/RConn1 -- -/RConn1 -- BCAM-/RConn1 -- DVL-/RConn1 -- GPS-/RConn1
  SSNR+/RConn1 -- Sonar Contactor/RConn1
  GPS+/RConn1 -- GPS Contactor/RConn1
  DVL Contactor/RConn1 -- DVL+/RConn1
  BCamera Contactor/RConn1 -- BCAM+/RConn1
  SPS1/RConn1 -- GPS Contactor/LConn1
  SPS2/RConn1 -- DVL Contactor/LConn1
  SPS3/RConn1 -- BCamera Contactor/LConn1
  SPS4/RConn1 -- Sonar Contactor/LConn1

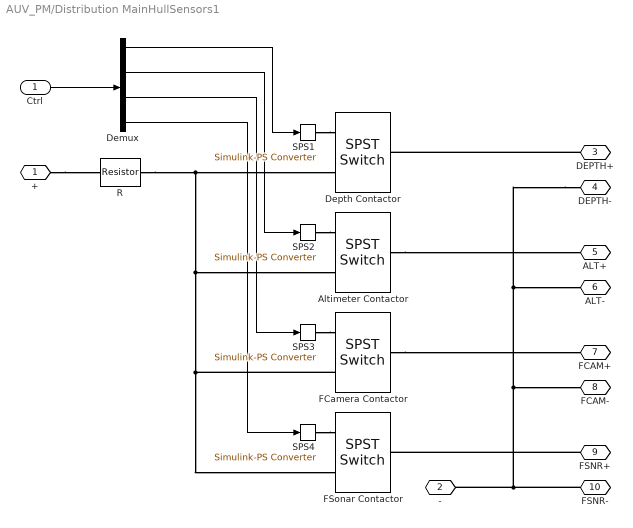
== system AUV_PM/Distribution MainHullSensors1 ==
  Ctrl : Inport
  Altimeter Contactor : ee_lib/Switches & Breakers/SPST Switch  R_closed=0.005 Ohm  G_open=1e-6 S  Threshold=0.5 V  Width=0 V  model_dynamics=0  t_on=1e-3 s  t_off=1e-3 s  initial_vT=0 V
      settings: SourceProductBaseCode=PS  InternalSimscapePortConfiguration="{\"Bottom\":[],\"Left\":[{\"id\":\"vT\",\"label\":\"vT\",\"type\":\"input\"},{\"id\":\"p\",\"label\":\"\",\"type\":\"foundation.electrical.electrical\"}],\"Right\":[{\"id\":\"n\",\"label\":\"\",\"type\":\"foundation.electrical.electrical\"}],\"Top\":[]}"
  Demux : Demux
  Depth Contactor : ee_lib/Switches & Breakers/SPST Switch  R_closed=0.005 Ohm  G_open=1e-6 S  Threshold=0.5 V  Width=0 V  model_dynamics=0  t_on=1e-3 s  t_off=1e-3 s  initial_vT=0 V
      settings: SourceProductBaseCode=PS  InternalSimscapePortConfiguration="{\"Bottom\":[],\"Left\":[{\"id\":\"vT\",\"label\":\"vT\",\"type\":\"input\"},{\"id\":\"p\",\"label\":\"\",\"type\":\"foundation.electrical.electrical\"}],\"Right\":[{\"id\":\"n\",\"label\":\"\",\"type\":\"foundation.electrical.electrical\"}],\"Top\":[]}"
  FCamera Contactor : ee_lib/Switches & Breakers/SPST Switch  R_closed=0.005 Ohm  G_open=1e-6 S  Threshold=0.5 V  Width=0 V  model_dynamics=0  t_on=1e-3 s  t_off=1e-3 s  initial_vT=0 V
      settings: SourceProductBaseCode=PS  InternalSimscapePortConfiguration="{\"Bottom\":[],\"Left\":[{\"id\":\"vT\",\"label\":\"vT\",\"type\":\"input\"},{\"id\":\"p\",\"label\":\"\",\"type\":\"foundation.electrical.electrical\"}],\"Right\":[{\"id\":\"n\",\"label\":\"\",\"type\":\"foundation.electrical.electrical\"}],\"Top\":[]}"
  FSonar Contactor : ee_lib/Switches & Breakers/SPST Switch  R_closed=0.005 Ohm  G_open=1e-6 S  Threshold=0.5 V  Width=0 V  model_dynamics=0  t_on=1e-3 s  t_off=1e-3 s  initial_vT=0 V
      settings: SourceProductBaseCode=PS  InternalSimscapePortConfiguration="{\"Bottom\":[],\"Left\":[{\"id\":\"vT\",\"label\":\"vT\",\"type\":\"input\"},{\"id\":\"p\",\"label\":\"\",\"type\":\"foundation.electrical.electrical\"}],\"Right\":[{\"id\":\"n\",\"label\":\"\",\"type\":\"foundation.electrical.electrical\"}],\"Top\":[]}"
  R : ee_lib/Passive/Resistor  R=0.005 Ohm  R_tol=5  enable_R_tol=0  tol_distribution=1  nSigma=4  enable_operating_limits=0  operating_limit_action=2  max_working_voltage=100 V  power_rating=1 W  enable_faults=0  fault_action=1  R_faulted=inf Ohm  enable_temporal_fault=0  t_fault=1 s  enable_behavioral_fault=0  max_permissible_current=1 A  t_fail_on_current=1 s  noise_mode=0  sample_time=1e-3 s  repeatability=1  auto_seed=2348838240  user_seed=0  Tdevice=25 degC  alpha=3.93e-3 1/K  Tmeas=25 degC  thermal_mass=100 J/K  power_derating_T1=70 degC  power_derating_T2=155 degC  operating_temperature_range_vec=[-50, 150] degC  temperature_specify=off  temperature_priority=High  temperature=298.15 K  temperature_nominal_specify=off  temperature_nominal_unit=K  temperature_nominal_value=1
  SPS{1..4} (4 alike) : nesl_utility/Simulink-PS Converter  PhysicalDomain=network_engine_domain  SubClassName=ps_input  LeftPortType=input  RightPortType=output  PseudoPeriodic=off  Frequencies=[]  NoiseDistribution=none  NoiseParameters=[]  Unit=1  AffineConversion=off  FilteringAndDerivatives=provide  SimscapeFilterOrder=1  InputFilterTimeConstant=0.001  UdotUserProvided=0
  + : PMIOPort  Side=Left
  - : PMIOPort  Port=2  Side=Left
  DEPTH+ : PMIOPort  Port=3  Side=Right
  DEPTH- : PMIOPort  Port=4  Side=Right
  ALT+ : PMIOPort  Port=5  Side=Right
  ALT- : PMIOPort  Port=6  Side=Right
  FCAM+ : PMIOPort  Port=7  Side=Right
  FCAM- : PMIOPort  Port=8  Side=Right
  FSNR+ : PMIOPort  Port=9  Side=Right
  FSNR- : PMIOPort  Port=10  Side=Right
  wires:
  Ctrl/1 -> Demux/1
  Demux/1 -> SPS1/1
  Demux/2 -> SPS2/1
  Demux/3 -> SPS3/1
  Demux/4 -> SPS4/1
  connections:
  SPS4/RConn1 -- FSonar Contactor/LConn1
  SPS3/RConn1 -- FCamera Contactor/LConn1
  SPS2/RConn1 -- Altimeter Contactor/LConn1
  SPS1/RConn1 -- Depth Contactor/LConn1
  FCamera Contactor/RConn1 -- FCAM+/RConn1
  Altimeter Contactor/RConn1 -- ALT+/RConn1
  DEPTH+/RConn1 -- Depth Contactor/RConn1
  FSNR+/RConn1 -- FSonar Contactor/RConn1
  DEPTH-/RConn1 -- ALT-/RConn1 -- FCAM-/RConn1 -- -/RConn1 -- FSNR-/RConn1
  +/RConn1 -- R/LConn1
  FCamera Contactor/LConn2 -- FSonar Contactor/LConn2 -- Altimeter Contactor/LConn2 -- Depth Contactor/LConn2 -- R/RConn1

== system AUV_PM/FCamera ==
  Electrical Reference3 : fl_lib/Electrical/Electrical Elements/Electrical Reference
      settings: SourceProductBaseCode=MT,SS
  R : ee_lib/Passive/Resistor  R=5 Ohm  R_tol=5  enable_R_tol=0  tol_distribution=1  nSigma=4  enable_operating_limits=0  operating_limit_action=2  max_working_voltage=100 V  power_rating=1 W  enable_faults=0  fault_action=1  R_faulted=inf Ohm  enable_temporal_fault=0  t_fault=1 s  enable_behavioral_fault=0  max_permissible_current=1 A  t_fail_on_current=1 s  noise_mode=0  sample_time=1e-3 s  repeatability=1  auto_seed=4112460543  user_seed=0  Tdevice=25 degC  alpha=3.93e-3 1/K  Tmeas=25 degC  thermal_mass=100 J/K  power_derating_T1=70 degC  power_derating_T2=155 degC  operating_temperature_range_vec=[-50, 150] degC  temperature_specify=off  temperature_priority=High  temperature=298.15 K  temperature_nominal_specify=off  temperature_nominal_unit=K  temperature_nominal_value=1
  + : PMIOPort  Side=Left
  - : PMIOPort  Port=2  Side=Left
  connections:
  -/RConn1 -- Electrical Reference3/LConn1 -- R/RConn1
  +/RConn1 -- R/LConn1

== system AUV_PM/Front Sonar ==
  Electrical Reference3 : fl_lib/Electrical/Electrical Elements/Electrical Reference
      settings: SourceProductBaseCode=MT,SS
  R : ee_lib/Passive/Resistor  R=5 Ohm  R_tol=5  enable_R_tol=0  tol_distribution=1  nSigma=4  enable_operating_limits=0  operating_limit_action=2  max_working_voltage=100 V  power_rating=1 W  enable_faults=0  fault_action=1  R_faulted=inf Ohm  enable_temporal_fault=0  t_fault=1 s  enable_behavioral_fault=0  max_permissible_current=1 A  t_fail_on_current=1 s  noise_mode=0  sample_time=1e-3 s  repeatability=1  auto_seed=4144164703  user_seed=0  Tdevice=25 degC  alpha=3.93e-3 1/K  Tmeas=25 degC  thermal_mass=100 J/K  power_derating_T1=70 degC  power_derating_T2=155 degC  operating_temperature_range_vec=[-50, 150] degC  temperature_specify=off  temperature_priority=High  temperature=298.15 K  temperature_nominal_specify=off  temperature_nominal_unit=K  temperature_nominal_value=1
  + : PMIOPort  Side=Left
  - : PMIOPort  Port=2  Side=Left
  connections:
  +/RConn1 -- R/LConn1
  R/RConn1 -- Electrical Reference3/LConn1 -- -/RConn1
